simulink model "simulacao_4_5"  (R2024a)
settings: Solver=VariableStepAuto  StartTime=0.0  StopTime=10.0  RelTol=1e-3
settings Model: Creator=alefp  LastModifiedBy=rodrigo
settings RTWCC: GPUComputeCapability=3.5

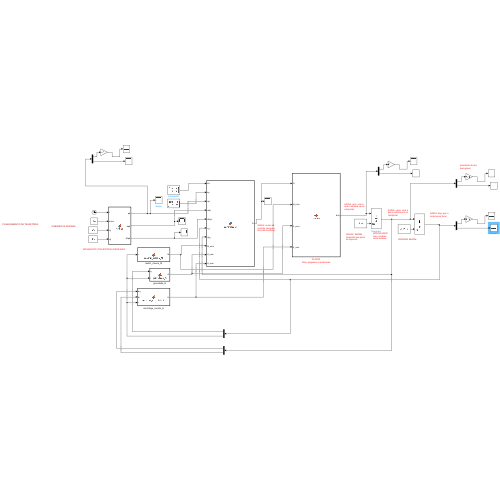
[thumbnail: Simulink's stored preview of the top-level diagram]
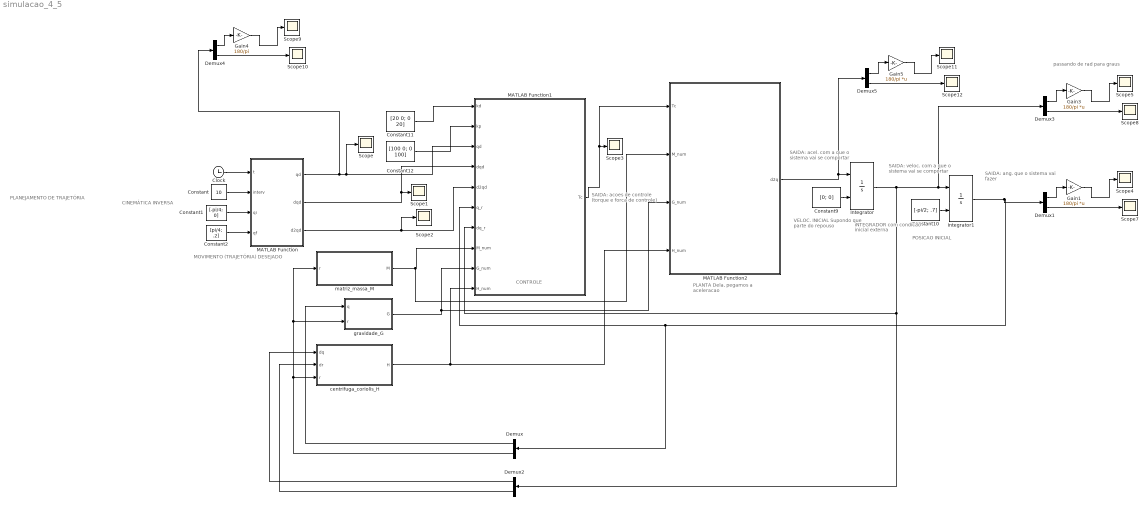
== system simulacao_4_5 ==
  note: MOVIMENTO (TRAJETÓRIA) DESEJADO
  note: CONTROLE
  note: PLANTA
      | Dela, pegamos a aceleracao
  note: INTEGRADOR
      | com condicao inicial externa
  note: VELOC. INICIAL
      | Supondo que parte do repouso
  note: POSICAO INICIAL
  note: SAIDA: ang. que o sistema vai fazer
  note: SAIDA: veloc. com a que o sistema vai se comportar
  note: SAIDA: acel. com a que o sistema vai se comportar
  note: SAIDA: acoes de controle (torque e forca de controle)
  note: passando de rad para graus
  note: PLANEJAMENTO DE TRAJETÓRIA
  note: CINEMÁTICA INVERSA
  Clock : Clock
  Constant : Constant  Value=10
  Constant1 : Constant  Value=[-pi/4; 0]
  Constant10 : Constant  Value=[-pi/2; .7]
  Constant11 : Constant  Value=[20 0; 0 20]
  Constant12 : Constant  Value=[100 0; 0 100]
  Constant2 : Constant  Value=[pi/4; .2]
  Constant9 : Constant  Value=[0; 0]
  Demux{,1..5} (6 alike) : Demux  Outputs=2
  Gain1 : Gain  Gain=180/pi  Multiplication=Matrix(K*u)
  Gain3 : Gain  Gain=180/pi  Multiplication=Matrix(K*u)
  Gain4 : Gain  Gain=180/pi
  Gain5 : Gain  Gain=180/pi  Multiplication=Matrix(K*u)
  Integrator : Integrator  InitialConditionSource=external
  Integrator1 : Integrator  InitialConditionSource=external
  MATLAB Function : MATLAB Function  TreatAsAtomicUnit=on
  MATLAB Function1 : MATLAB Function  TreatAsAtomicUnit=on
  MATLAB Function2 : MATLAB Function  TreatAsAtomicUnit=on
  Scope{,1..5,7..12} (12 alike) : Scope
  centrifuga_coriolis_H : MATLAB Function  TreatAsAtomicUnit=on
  gravidade_G : MATLAB Function  TreatAsAtomicUnit=on
  matriz_massa_M : MATLAB Function  TreatAsAtomicUnit=on
  wires:
  MATLAB Function/2(dqd) -> Scope1/1, MATLAB Function1/4(dqd)
  MATLAB Function/3(d2qd) -> Scope2/1, MATLAB Function1/5(d2qd)
  MATLAB Function/1(qd) -> Demux4/1, MATLAB Function1/3(qd), Scope/1
  Constant/1 -> MATLAB Function/2(interv)
  Constant1/1 -> MATLAB Function/3(qi)
  Clock/1 -> MATLAB Function/1(t)
  Constant2/1 -> MATLAB Function/4(qf)
  MATLAB Function1/1(Tc) -> Scope3/1, MATLAB Function2/1(Tc)
  Constant9/1 -> Integrator/2
  Constant10/1 -> Integrator1/2
  Integrator/1 -> Demux2/1, MATLAB Function1/7(dq_r), Demux3/1, Integrator1/1
  Integrator1/1 -> Demux1/1, Demux/1, MATLAB Function1/6(q_r)
  Constant11/1 -> MATLAB Function1/1(kd)
  Constant12/1 -> MATLAB Function1/2(kp)
  Demux1/2 -> Scope7/1
  Gain1/1 -> Scope4/1
  Demux1/1 -> Gain1/1
  Demux4/1 -> Gain4/1
  Gain4/1 -> Scope9/1
  Demux4/2 -> Scope10/1
  Demux3/1 -> Gain3/1
  Gain3/1 -> Scope5/1
  Demux3/2 -> Scope8/1
  Demux5/1 -> Gain5/1
  Gain5/1 -> Scope11/1
  Demux5/2 -> Scope12/1
  MATLAB Function2/1(d2q) -> Demux5/1, Integrator/1
  matriz_massa_M/1(M) -> MATLAB Function2/2(M_num), MATLAB Function1/8(M_num)
  gravidade_G/1(G) -> MATLAB Function2/3(G_num), MATLAB Function1/9(G_num)
  centrifuga_coriolis_H/1(H) -> MATLAB Function2/4(H_num), MATLAB Function1/10(H_num)
  Demux/1 -> gravidade_G/1(q)
  Demux/2 -> matriz_massa_M/1(r), gravidade_G/2(r), centrifuga_coriolis_H/3(r)
  Demux2/1 -> centrifuga_coriolis_H/1(dq)
  Demux2/2 -> centrifuga_coriolis_H/2(dr)

== matlab function simulacao_4_5/MATLAB Function1 ==
  data: kd input; kp input; qd input; dqd input; d2qd input; q_r input; dq_r input; M_num input; G_num input; H_num input; Tc output
function Tc  = controlador(kd, kp, qd, dqd, d2qd, q_r, dq_r, M_num, G_num, H_num)

Tc = M_num*(d2qd + kd*(dqd-dq_r) + kp*(qd-q_r)) + H_num + G_num;

== matlab function simulacao_4_5/MATLAB Function ==
  data: t input; qd output; interv input; qi input; qf input; dqd output; d2qd output
function [qd, dqd, d2qd] = cinCub(t, interv, qi, qf)

tf = interv;
A = [1 0 0 0; 0 1 0 0; 1 tf tf^2 tf^3; 0 1 2*tf 3*tf^2];
b = [qi(1); 0; qf(1); 0];
x = inv(A)*b;

qd = zeros(2,1);
dqd = qd;
d2qd = qd;


qd(1,1) = x(1) + x(2)*t + x(3)*t^2 + x(4)*t^3;
dqd(1,1) = x(2) + 2*x(3)*t + 3*x(4)*t^2;
d2qd(1,1) = 2*x(3) + 6*x(4)*t;


b = [qi(2); 0; qf(2); 0];
x = inv(A)*b;

qd(2,1) = x(1) + x(2)*t + x(3)*t^2 + x(4)*t^3;
dqd(2,1) = x(2) + 2*x(3)*t + 3*x(4)*t^2;
d2qd(2,1) = 2*x(3) + 6*x(4)*t;

== matlab function simulacao_4_5/MATLAB Function2 ==
  data: d2q output; Tc input; M_num input; G_num input; H_num input
function d2q  = planta(Tc, M_num, G_num, H_num) % a planta devolve a aceleração simulada 


d2q = M_num\(Tc-H_num-G_num); % A\B == inv(A)*B

== matlab function simulacao_4_5/matriz_massa_M ==
  data: r input; M output
function M = matriz_massa_M(r)
%#codegen

%    This function was generated by the Symbolic Math Toolbox version 24.1.
%    05-Sep-2024 22:50:15

% r = complex(r);  % if required to enforce complex operations
M = reshape([r.^2.*5.0+2.677083333333333e+1,0.0,0.0,5.0],[2,2]);
end

== matlab function simulacao_4_5/gravidade_G ==
  data: q input; G output; r input
function G = gravidade_G(q,r)
%#codegen

%    This function was generated by the Symbolic Math Toolbox version 24.1.
%    05-Sep-2024 22:50:16

% q = complex(q);  % if required to enforce complex operations
% r = complex(r);  % if required to enforce complex operations
G = [cos(q).*(r.*1.0e+1+4.0e+1).*(9.81e+2./2.0e+2);sin(q).*(9.81e+2./2.0e+1)];
end

== matlab function simulacao_4_5/centrifuga_coriolis_H ==
  data: dq input; H output; dr input; r input
function H = centrifuga_coriolis_H(dq,dr,r)
%#codegen

%    This function was generated by the Symbolic Math Toolbox version 24.1.
%    05-Sep-2024 22:50:16

% dq = complex(dq);  % if required to enforce complex operations
% dr = complex(dr);  % if required to enforce complex operations
% r = complex(r);  % if required to enforce complex operations
H = [dq.*dr.*r.*1.0e+1;dq.^2.*r.*-5.0];
end
